simulink model "hcu_main_ADASwEPS"  (Simulink 8.2)
settings: Solver=FixedStepDiscrete  StartTime=0.0  StopTime=inf  FixedStep=0.001  RelTol=1e-3
PostLoadFcn:
  | , if any(exist('dsrtsu_mdlpostloadfcn', 'file') == [2, 3, 6]), try dsrtsu_mdlpostloadfcn('Execute', bdroot); catch fprintf('Error in PostLoadFcn (dsrtsu_mdlpostloadfcn) for model "%s":\n %s\n', bdroot, lasterr); end, end,
values from neighbouring files (symbols this model uses):
  C_TASK_1MS_S = (	C_TICK_TIME_S       )    [hcu_local_hdr.m]    (also in temp_ovrd_values.m = double(	0.001                  ))
  C_TICK_TIME_S = single(	0.005	    	)    [hcu_local_hdr.m]
  ENUM_EPSLFCSTATUS_ACTIVE = uint8(  2  )    [hcu_local_hdr.m]
  ENUM_EPSLFCSTATUS_TRANSITION = uint8(  3  )    [hcu_local_hdr.m]
  ENUM_EPSLKASTATUS_ACTIVE = uint8(  2  )    [hcu_local_hdr.m]
  ENUM_EPSMODEREQ_ANGLE = uint8(  1  )    [hcu_local_hdr.m]
  ENUM_EPSMODEREQ_INTERNAL = uint8(  0  )    [hcu_local_hdr.m]
  ENUM_EPSMODEREQ_TORQUE = uint8(  2  )    [hcu_local_hdr.m]
  ENUM_GEARPOSN_1ST = uint8(  1  )    [hcu_local_hdr.m]
  ENUM_GEARPOSN_2ND = uint8(  2  )    [hcu_local_hdr.m]
  ENUM_GEARPOSN_3RD = uint8(  3  )    [hcu_local_hdr.m]
  ENUM_GEARPOSN_4TH = uint8(  4  )    [hcu_local_hdr.m]
  ENUM_GEARPOSN_5TH = uint8(  5  )    [hcu_local_hdr.m]
  ENUM_GEARPOSN_6TH = uint8(  6  )    [hcu_local_hdr.m]
  ENUM_GEARPOSN_R = uint8(  7  )    [hcu_local_hdr.m]
  FALSE = boolean( 0 )    [hcu_local_hdr.m]
  TRUE = boolean( 1 )    [hcu_local_hdr.m]
undefined symbols (not defined in the file or in its folder): AISP_EPSCurrent_pct, AISP_TqASensorDelta_pct, AISP_TqBSensorDelta_pct, dHAL_IN, hal, INVALID_ABS1_TIMEOUT, INVALID_ABS2_TIMEOUT, INVALID_ABS3_TIMEOUT, INVALID_ABS4_TIMEOUT, INVALID_AC1_TIMEOUT, INVALID_ADASTORQ_REQ, INVALID_BCM1_TIMEOUT, INVALID_BCM2_TIMEOUT, INVALID_BOOSTER_VAC, INVALID_CSW1_TIMEOUT, INVALID_CUR_VEHDECE, INVALID_CURBRAKEDECE_REQ, INVALID_CURSTEERANG_REQ, INVALID_CURSTEERTQ_REQ, INVALID_ECM1_TIMEOUT, INVALID_ECM2_TIMEOUT, INVALID_ECM3_TIMEOUT, INVALID_ECM9_TIMEOUT, INVALID_ENG_TORQUE_FRICTIONAL, INVALID_ENG_TORQUE_INDICATED, INVALID_ENG_TORQUE_INDICATEDCOR, INVALID_ENG_TQ_MAX, INVALID_ENG_TQ_MIN, INVALID_EPAS2_TIMEOUT, INVALID_EPAS3_TIMEOUT, INVALID_EPB1_TIMEOUT, INVALID_EPS_BATTVOLT, INVALID_ESC_BATTVOLT, INVALID_GRADE, INVALID_HCU3_TIMEOUT, INVALID_HCU4_TIMEOUT, INVALID_HMI1_TIMEOUT, INVALID_HMI2_TIMEOUT, INVALID_LAT_ACC, INVALID_LONG_ACC, INVALID_MC_PRESSURE, INVALID_METER1_TIMEOUT, INVALID_METER3_TIMEOUT, INVALID_METER_VEHSPD, INVALID_ODO_METER, INVALID_OUTSIDE_TEMP, INVALID_PARKBRAKEBIND_STAT, INVALID_PEDALTQ_REQ, INVALID_SAS1_TIMEOUT, INVALID_SAS_ANGLE, INVALID_SHIFTER_POSN, INVALID_TCM1_TIMEOUT, INVALID_TCM2_TIMEOUT, INVALID_VCU1_TIMEOUT, INVALID_VCU2_TIMEOUT, INVALID_VEH_CRASH, INVALID_VEH_SPD, INVALID_WHEEL_SPD, INVALID_YAW_RATE, KHAL_MssgIdObj1_num ... (+8)
libraries: simulink x147, hcu_lib x38, rti1401lib_dio_type3 x4, rtimmsu_dsrtlib x3, app x1, rtiethernetudplib x1, rti1401lib_adc_type4 x1, rti1401lib_dac_type3 x1, inp x1, lidr x1, outp x1
(part 14 of 15)

== system hcu_main_ADASwEPS/dHAL_IN/HAL_IN_VCU/BO__1361_VCU2__8_VCU/ChecksumCalculation ==
  CAN1_Rx : Inport
  Add : Sum  Inputs=16
  Bitwise Operator : simulink/Logic and Bit Operations/Bitwise Operator  logicop=XOR  UseBitMask=off  NumInputPorts=2  BitMask=bin2dec('11011001')  BitMaskRealWorld=Stored Integer
  Bus Selector : BusSelector  OutputSignals=VCU2.RAW_Byte_1,VCU2.RAW_Byte_2,VCU2.RAW_Byte_3,VCU2.RAW_Byte_4,VCU2.RAW_Byte_5,VCU2.RAW_Byte_6,VCU2.RAW_Byte_7,VCU2.RAW_Byte_8,VCU2.VCU2_LifeCount
  Constant1 : Constant  Value=hex2dec('10')  OutDataTypeStr=uint8
  Constant2 : Constant  Value=hex2dec('ff')  OutDataTypeStr=uint8
  Data Type Conversion{,1..23} (24 alike) : DataTypeConversion  OutDataTypeStr=uint8
  Extract Bits{1,3,5,7,9,12,14} (7 alike) : simulink/Logic and Bit Operations/Extract Bits  bitsToExtract=Lower half  numBits=8  bitIdxRange=[0 7]  outScalingMode=Preserve fixed-point scaling
  Extract Bits{2,4,6,8,10..11,13,15} (8 alike) : simulink/Logic and Bit Operations/Extract Bits  bitsToExtract=Upper half  numBits=8  bitIdxRange=[0 7]  outScalingMode=Preserve fixed-point scaling
  Math Function : Math  Operator=mod  SaturateOnIntegerOverflow=on
  Shift Arithmetic{,1..7} (8 alike) : ArithShift  BitShiftNumber=4
  Message_Checksum : Outport
  wires:
  Bus Selector/1 -> Data Type Conversion/1  "<RAW_Byte_1>"
  Extract Bits2/1 -> Data Type Conversion1/1
  Extract Bits1/1 -> Data Type Conversion2/1
  Data Type Conversion1/1 -> Shift Arithmetic/1
  Data Type Conversion/1 -> Extract Bits2/1, Extract Bits1/1
  Extract Bits4/1 -> Data Type Conversion4/1
  Extract Bits3/1 -> Data Type Conversion5/1
  Data Type Conversion4/1 -> Shift Arithmetic1/1
  Data Type Conversion3/1 -> Extract Bits3/1, Extract Bits4/1
  Shift Arithmetic/1 -> Add/1
  Data Type Conversion2/1 -> Add/2
  Shift Arithmetic1/1 -> Add/3
  Data Type Conversion5/1 -> Add/4
  Bus Selector/2 -> Data Type Conversion3/1  "<RAW_Byte_2>"
  Extract Bits6/1 -> Data Type Conversion7/1
  Extract Bits5/1 -> Data Type Conversion8/1
  Data Type Conversion7/1 -> Shift Arithmetic2/1
  Data Type Conversion6/1 -> Extract Bits6/1, Extract Bits5/1
  Shift Arithmetic2/1 -> Add/5
  Data Type Conversion8/1 -> Add/6
  Bus Selector/3 -> Data Type Conversion6/1  "<RAW_Byte_3>"
  Extract Bits8/1 -> Data Type Conversion10/1
  Extract Bits7/1 -> Data Type Conversion11/1
  Data Type Conversion10/1 -> Shift Arithmetic3/1
  Data Type Conversion9/1 -> Extract Bits7/1, Extract Bits8/1
  Shift Arithmetic3/1 -> Add/7
  Data Type Conversion11/1 -> Add/8
  Bus Selector/4 -> Data Type Conversion9/1  "<RAW_Byte_4>"
  Extract Bits10/1 -> Data Type Conversion12/1
  Extract Bits9/1 -> Data Type Conversion13/1
  Data Type Conversion12/1 -> Shift Arithmetic4/1
  Data Type Conversion14/1 -> Extract Bits10/1, Extract Bits9/1
  Shift Arithmetic4/1 -> Add/9
  Data Type Conversion13/1 -> Add/10
  Bus Selector/5 -> Data Type Conversion14/1  "<RAW_Byte_5>"
  Extract Bits11/1 -> Data Type Conversion15/1
  Extract Bits12/1 -> Data Type Conversion16/1
  Data Type Conversion15/1 -> Shift Arithmetic5/1
  Data Type Conversion17/1 -> Extract Bits12/1, Extract Bits11/1
  Shift Arithmetic5/1 -> Add/11
  Data Type Conversion16/1 -> Add/12
  Bus Selector/6 -> Data Type Conversion17/1  "<RAW_Byte_6>"
  Extract Bits13/1 -> Data Type Conversion18/1
  Extract Bits14/1 -> Data Type Conversion19/1
  Data Type Conversion18/1 -> Shift Arithmetic6/1
  Data Type Conversion20/1 -> Extract Bits13/1, Extract Bits14/1
  Shift Arithmetic6/1 -> Add/13
  Data Type Conversion19/1 -> Add/14
  Bus Selector/7 -> Data Type Conversion20/1  "<RAW_Byte_7>"
  Extract Bits15/1 -> Data Type Conversion21/1
  Data Type Conversion21/1 -> Shift Arithmetic7/1
  Data Type Conversion23/1 -> Extract Bits15/1
  Shift Arithmetic7/1 -> Add/15
  Bus Selector/8 -> Data Type Conversion23/1  "<RAW_Byte_8>"
  Data Type Conversion22/1 -> Add/16
  Add/1 -> Bitwise Operator/1
  Constant2/1 -> Bitwise Operator/2
  Bitwise Operator/1 -> Math Function/1
  Constant1/1 -> Math Function/2
  Math Function/1 -> Message_Checksum/1
  CAN1_Rx/1 -> Bus Selector/1
  Bus Selector/9 -> Data Type Conversion22/1  "<VCU2_LifeCount>"

== system hcu_main_ADASwEPS/dHAL_IN/dHAL_IN_ABS/BO_864_ABS2_8_ABS/ChecksumCalculation ==
  CAN1_Rx : Inport
  Add : Sum  Inputs=16
  Bitwise Operator : simulink/Logic and Bit Operations/Bitwise Operator  logicop=XOR  UseBitMask=off  NumInputPorts=2  BitMask=bin2dec('11011001')  BitMaskRealWorld=Stored Integer
  Bus Selector : BusSelector  OutputSignals=ABS2.RAW_Byte_1,ABS2.RAW_Byte_2,ABS2.RAW_Byte_3,ABS2.RAW_Byte_4,ABS2.RAW_Byte_5,ABS2.RAW_Byte_6,ABS2.RAW_Byte_7,ABS2.RAW_Byte_8
  Constant : Constant  Value=uint8(2)
  Constant1 : Constant  Value=hex2dec('10')  OutDataTypeStr=uint8
  Constant2 : Constant  Value=hex2dec('ff')  OutDataTypeStr=uint8
  Data Type Conversion{,1..21,23} (23 alike) : DataTypeConversion  OutDataTypeStr=uint8
  Extract Bits{1,3,5,7,9,12,14} (7 alike) : simulink/Logic and Bit Operations/Extract Bits  bitsToExtract=Lower half  numBits=8  bitIdxRange=[0 7]  outScalingMode=Preserve fixed-point scaling
  Extract Bits{2,4,6,8,10..11,13,15} (8 alike) : simulink/Logic and Bit Operations/Extract Bits  bitsToExtract=Upper half  numBits=8  bitIdxRange=[0 7]  outScalingMode=Preserve fixed-point scaling
  Math Function : Math  Operator=mod  SaturateOnIntegerOverflow=on
  Shift Arithmetic{,1..7} (8 alike) : ArithShift  BitShiftNumber=4
  Message_Checksum : Outport
  wires:
  Bus Selector/1 -> Data Type Conversion/1  "<RAW_Byte_1>"
  Extract Bits2/1 -> Data Type Conversion1/1
  Extract Bits1/1 -> Data Type Conversion2/1
  Data Type Conversion1/1 -> Shift Arithmetic/1
  Data Type Conversion/1 -> Extract Bits2/1, Extract Bits1/1
  Extract Bits4/1 -> Data Type Conversion4/1
  Extract Bits3/1 -> Data Type Conversion5/1
  Data Type Conversion4/1 -> Shift Arithmetic1/1
  Data Type Conversion3/1 -> Extract Bits3/1, Extract Bits4/1
  Shift Arithmetic/1 -> Add/1
  Data Type Conversion2/1 -> Add/2
  Shift Arithmetic1/1 -> Add/3
  Data Type Conversion5/1 -> Add/4
  Bus Selector/2 -> Data Type Conversion3/1  "<RAW_Byte_2>"
  Extract Bits6/1 -> Data Type Conversion7/1
  Extract Bits5/1 -> Data Type Conversion8/1
  Data Type Conversion7/1 -> Shift Arithmetic2/1
  Data Type Conversion6/1 -> Extract Bits6/1, Extract Bits5/1
  Shift Arithmetic2/1 -> Add/5
  Data Type Conversion8/1 -> Add/6
  Bus Selector/3 -> Data Type Conversion6/1  "<RAW_Byte_3>"
  Extract Bits8/1 -> Data Type Conversion10/1
  Extract Bits7/1 -> Data Type Conversion11/1
  Data Type Conversion10/1 -> Shift Arithmetic3/1
  Data Type Conversion9/1 -> Extract Bits7/1, Extract Bits8/1
  Shift Arithmetic3/1 -> Add/7
  Data Type Conversion11/1 -> Add/8
  Bus Selector/4 -> Data Type Conversion9/1  "<RAW_Byte_4>"
  Extract Bits10/1 -> Data Type Conversion12/1
  Extract Bits9/1 -> Data Type Conversion13/1
  Data Type Conversion12/1 -> Shift Arithmetic4/1
  Data Type Conversion14/1 -> Extract Bits10/1, Extract Bits9/1
  Shift Arithmetic4/1 -> Add/9
  Data Type Conversion13/1 -> Add/10
  Bus Selector/5 -> Data Type Conversion14/1  "<RAW_Byte_5>"
  Extract Bits11/1 -> Data Type Conversion15/1
  Extract Bits12/1 -> Data Type Conversion16/1
  Data Type Conversion15/1 -> Shift Arithmetic5/1
  Data Type Conversion17/1 -> Extract Bits12/1, Extract Bits11/1
  Shift Arithmetic5/1 -> Add/11
  Data Type Conversion16/1 -> Add/12
  Bus Selector/6 -> Data Type Conversion17/1  "<RAW_Byte_6>"
  Extract Bits13/1 -> Data Type Conversion18/1
  Extract Bits14/1 -> Data Type Conversion19/1
  Data Type Conversion18/1 -> Shift Arithmetic6/1
  Data Type Conversion20/1 -> Extract Bits13/1, Extract Bits14/1
  Shift Arithmetic6/1 -> Add/13
  Data Type Conversion19/1 -> Add/14
  Bus Selector/7 -> Data Type Conversion20/1  "<RAW_Byte_7>"
  Extract Bits15/1 -> Data Type Conversion21/1
  Data Type Conversion21/1 -> Shift Arithmetic7/1
  Data Type Conversion23/1 -> Extract Bits15/1
  Shift Arithmetic7/1 -> Add/15
  Bus Selector/8 -> Data Type Conversion23/1  "<RAW_Byte_8>"
  Constant/1 -> Add/16
  Add/1 -> Bitwise Operator/1
  Constant2/1 -> Bitwise Operator/2
  Bitwise Operator/1 -> Math Function/1
  Constant1/1 -> Math Function/2
  Math Function/1 -> Message_Checksum/1
  CAN1_Rx/1 -> Bus Selector/1

== system hcu_main_ADASwEPS/dHAL_IN/dHAL_IN_EPAS/BO__1365_EPAS3__8_EPAS/ChecksumCalculation ==
  EPAS3_LifeCount : Inport
  CAN1_Rx : Inport  Port=2
  Bitwise Operator1 : simulink/Logic and Bit Operations/Bitwise Operator  logicop=XOR  UseBitMask=off  NumInputPorts=7  BitMask=bin2dec('11011001')  BitMaskRealWorld=Stored Integer
  Bitwise Operator2 : simulink/Logic and Bit Operations/Bitwise Operator  logicop=XOR  UseBitMask=off  NumInputPorts=3  BitMask=bin2dec('11011001')  BitMaskRealWorld=Stored Integer
  Bus Selector : BusSelector  OutputSignals=EPAS3.RAW_Byte_1,EPAS3.RAW_Byte_2,EPAS3.RAW_Byte_3,EPAS3.RAW_Byte_4,EPAS3.RAW_Byte_5,EPAS3.RAW_Byte_6,EPAS3.RAW_Byte_7
  Data Type Conversion{1..10} (10 alike) : DataTypeConversion  OutDataTypeStr=uint8
  Extract Bits5 : simulink/Logic and Bit Operations/Extract Bits  bitsToExtract=Lower half  numBits=8  bitIdxRange=[0 7]  outScalingMode=Preserve fixed-point scaling
  Extract Bits6 : simulink/Logic and Bit Operations/Extract Bits  bitsToExtract=Upper half  numBits=8  bitIdxRange=[0 7]  outScalingMode=Preserve fixed-point scaling
  Shift Arithmetic2 : ArithShift  BitShiftNumber=4
  Message_Checksum : Outport
  wires:
  [CAN1_Rx] -> Bus Selector/1
  CAN1_Rx/1 -> [CAN1_Rx]
  Bitwise Operator2/1 -> Message_Checksum/1
  EPAS3_LifeCount/1 -> Data Type Conversion10/1
  Data Type Conversion8/1 -> Bitwise Operator2/2
  Shift Arithmetic2/1 -> Bitwise Operator2/1
  Bitwise Operator1/1 -> Extract Bits5/1, Extract Bits6/1
  Data Type Conversion9/1 -> Bitwise Operator1/4
  Data Type Conversion6/1 -> Bitwise Operator1/3
  Data Type Conversion3/1 -> Bitwise Operator1/2
  Data Type Conversion1/1 -> Bitwise Operator1/1
  Bus Selector/1 -> Data Type Conversion1/1  "<RAW_Byte_1>"
  Bus Selector/4 -> Data Type Conversion9/1  "<RAW_Byte_4>"
  Bus Selector/3 -> Data Type Conversion6/1  "<RAW_Byte_3>"
  Data Type Conversion7/1 -> Shift Arithmetic2/1
  Extract Bits5/1 -> Data Type Conversion8/1
  Extract Bits6/1 -> Data Type Conversion7/1
  Bus Selector/2 -> Data Type Conversion3/1  "<RAW_Byte_2>"
  Data Type Conversion2/1 -> Bitwise Operator1/5
  Data Type Conversion4/1 -> Bitwise Operator1/6
  Data Type Conversion5/1 -> Bitwise Operator1/7
  Bus Selector/5 -> Data Type Conversion2/1  "<RAW_Byte_5>"
  Bus Selector/6 -> Data Type Conversion4/1  "<RAW_Byte_6>"
  Bus Selector/7 -> Data Type Conversion5/1  "<RAW_Byte_7>"
  Data Type Conversion10/1 -> Bitwise Operator2/3

== system hcu_main_ADASwEPS/dHAL_IN/dHAL_IN_EPAS/BO__922_SAS1__8_EPAS/ChecksumCalculation ==
  SAS_MsgCount : Inport
  CAN1_Rx : Inport  Port=2
  Bitwise Operator1 : simulink/Logic and Bit Operations/Bitwise Operator  logicop=XOR  UseBitMask=off  NumInputPorts=4  BitMask=bin2dec('11011001')  BitMaskRealWorld=Stored Integer
  Bitwise Operator2 : simulink/Logic and Bit Operations/Bitwise Operator  logicop=XOR  UseBitMask=off  NumInputPorts=3  BitMask=bin2dec('11011001')  BitMaskRealWorld=Stored Integer
  Bus Selector : BusSelector  OutputSignals=SAS1.RAW_Byte_1,SAS1.RAW_Byte_2,SAS1.RAW_Byte_3,SAS1.RAW_Byte_4
  Data Type Conversion{1..3,6..9} (7 alike) : DataTypeConversion  OutDataTypeStr=uint8
  Extract Bits5 : simulink/Logic and Bit Operations/Extract Bits  bitsToExtract=Lower half  numBits=8  bitIdxRange=[0 7]  outScalingMode=Preserve fixed-point scaling
  Extract Bits6 : simulink/Logic and Bit Operations/Extract Bits  bitsToExtract=Upper half  numBits=8  bitIdxRange=[0 7]  outScalingMode=Preserve fixed-point scaling
  Shift Arithmetic2 : ArithShift  BitShiftNumber=4
  Message_Checksum : Outport
  wires:
  Bus Selector/2 -> Data Type Conversion3/1  "<RAW_Byte_2>"
  Extract Bits6/1 -> Data Type Conversion7/1
  Extract Bits5/1 -> Data Type Conversion8/1
  Data Type Conversion7/1 -> Shift Arithmetic2/1
  Bus Selector/3 -> Data Type Conversion6/1  "<RAW_Byte_3>"
  Bus Selector/4 -> Data Type Conversion9/1  "<RAW_Byte_4>"
  Bus Selector/1 -> Data Type Conversion1/1  "<RAW_Byte_1>"
  Data Type Conversion1/1 -> Bitwise Operator1/1
  Data Type Conversion3/1 -> Bitwise Operator1/2
  Data Type Conversion6/1 -> Bitwise Operator1/3
  Data Type Conversion9/1 -> Bitwise Operator1/4
  Bitwise Operator1/1 -> Extract Bits6/1, Extract Bits5/1
  Shift Arithmetic2/1 -> Bitwise Operator2/1
  Data Type Conversion8/1 -> Bitwise Operator2/2
  SAS_MsgCount/1 -> Data Type Conversion2/1
  Bitwise Operator2/1 -> Message_Checksum/1
  CAN1_Rx/1 -> Bus Selector/1
  Data Type Conversion2/1 -> Bitwise Operator2/3

== system hcu_main_ADASwEPS/dHAL_IN/dHAL_IN_EPAS/BO__926_EPAS2__8_EPAS/ChecksumCalculation ==
  SAS_MsgCount : Inport
  CAN1_Rx : Inport  Port=2
  Bitwise Operator1 : simulink/Logic and Bit Operations/Bitwise Operator  logicop=XOR  UseBitMask=off  NumInputPorts=5  BitMask=bin2dec('11011001')  BitMaskRealWorld=Stored Integer
  Bitwise Operator2 : simulink/Logic and Bit Operations/Bitwise Operator  logicop=XOR  UseBitMask=off  NumInputPorts=3  BitMask=bin2dec('11011001')  BitMaskRealWorld=Stored Integer
  Bus Selector : BusSelector  OutputSignals=EPAS2.RAW_Byte_1,EPAS2.RAW_Byte_2,EPAS2.RAW_Byte_3,EPAS2.RAW_Byte_4,EPAS2.RAW_Byte_5
  Data Type Conversion{1..4,6..9} (8 alike) : DataTypeConversion  OutDataTypeStr=uint8
  Extract Bits5 : simulink/Logic and Bit Operations/Extract Bits  bitsToExtract=Lower half  numBits=8  bitIdxRange=[0 7]  outScalingMode=Preserve fixed-point scaling
  Extract Bits6 : simulink/Logic and Bit Operations/Extract Bits  bitsToExtract=Upper half  numBits=8  bitIdxRange=[0 7]  outScalingMode=Preserve fixed-point scaling
  Shift Arithmetic2 : ArithShift  BitShiftNumber=4
  Message_Checksum : Outport
  wires:
  Bus Selector/2 -> Data Type Conversion3/1  "<RAW_Byte_2>"
  Extract Bits6/1 -> Data Type Conversion7/1
  Extract Bits5/1 -> Data Type Conversion8/1
  Data Type Conversion7/1 -> Shift Arithmetic2/1
  Bus Selector/3 -> Data Type Conversion6/1  "<RAW_Byte_3>"
  Bus Selector/4 -> Data Type Conversion9/1  "<RAW_Byte_4>"
  Bus Selector/1 -> Data Type Conversion1/1  "<RAW_Byte_1>"
  Data Type Conversion1/1 -> Bitwise Operator1/1
  Data Type Conversion3/1 -> Bitwise Operator1/2
  Data Type Conversion6/1 -> Bitwise Operator1/3
  Data Type Conversion9/1 -> Bitwise Operator1/4
  Bitwise Operator1/1 -> Extract Bits5/1, Extract Bits6/1
  Shift Arithmetic2/1 -> Bitwise Operator2/1
  Data Type Conversion8/1 -> Bitwise Operator2/2
  SAS_MsgCount/1 -> Data Type Conversion4/1
  Bitwise Operator2/1 -> Message_Checksum/1
  CAN1_Rx/1 -> [CAN1_Rx]
  [CAN1_Rx] -> Bus Selector/1
  Bus Selector/5 -> Data Type Conversion2/1  "<RAW_Byte_5>"
  Data Type Conversion2/1 -> Bitwise Operator1/5
  Data Type Conversion4/1 -> Bitwise Operator2/3

== system hcu_main_ADASwEPS/EPSS/EPSS/AngleMode/Angle2Torque/Hysteresis (higher limit) ==
  Input : Inport
  Switch_on_point : Inport  Port=2
  Switch_off_point : Inport  Port=3
  Data Type Conversion : DataTypeConversion
  Logical Operator1 : Logic  AllPortsSameDT=off  OutDataTypeStr=boolean
  Logical Operator2 : Logic  Operator=NOT  AllPortsSameDT=off  OutDataTypeStr=boolean
  Logical Operator3 : Logic  Operator=OR  AllPortsSameDT=off  OutDataTypeStr=boolean
  Relational Operator : RelationalOperator  OutDataTypeStr=boolean
  Relational Operator1 : RelationalOperator  Operator=<=  OutDataTypeStr=boolean
  Unit Delay : UnitDelay  SampleTime=-1
  Output : Outport
  wires:
  Switch_on_point/1 -> Relational Operator/2
  Switch_off_point/1 -> Relational Operator1/2
  Logical Operator2/1 -> Logical Operator1/2
  Logical Operator1/1 -> Unit Delay/1, Data Type Conversion/1
  Unit Delay/1 -> Logical Operator3/1
  Input/1 -> Relational Operator/1, Relational Operator1/1
  Relational Operator/1 -> Logical Operator3/2
  Logical Operator3/1 -> Logical Operator1/1
  Relational Operator1/1 -> Logical Operator2/1
  Data Type Conversion/1 -> Output/1

== system hcu_main_ADASwEPS/EPSS/EPSS/AngleMode/Angle2Torque/InverseAssistTable ==
  VEPSS_MotPWMReqAngle_pct : Inport
  VDINR_VehSpd_kph : Inport  Port=2
  MEPSS_EPSMotPWMRescalingInv_pct : Lookup  InputValues=[-250 -3 0 3 250]  Table=[-100 -3 0 3 100]  LookUpMeth=Interpolation-Use End Values
      settings: AttributesFormatString="Input=\"%<InputValues>\"\\nOutput=\"%<Table>\""
  MEPSS_TqAssistPWM_pct : Lookup  InputValues="[-100\t-95\t-90\t-85\t-80\t-75\t-70\t-65\t-60\t-55\t-50\t-45\t-40\t-35\t-30\t-25\t-20\t-15\t-10\t-5\t0\t5\t10\t15\t20\t25\t30\t35\t40\t45\t50\t55\t60\t65\t70\t75\t80\t85\t90\t95\t100]"  Table=[-10:0.5:10]  LookUpMeth=Interpolation-Use End Values
      settings: AttributesFormatString="Input=\"%<InputValues>\"\\nOutput=\"%<Table>\""
  MEPSS_VehSpdPWMMult_rat : Lookup  InputValues=[-100 -80 -60 -40 -20 -10 0 10 20 40 60 80 100]  Table=[1 1 1 1 1 1 1 1 1 1 1 1 1]  LookUpMeth=Interpolation-Use End Values
      settings: AttributesFormatString="Input=\"%<InputValues>\"\\nOutput=\"%<Table>\""
  Product : Product  Inputs=*/
  VEPSS_StrWhlTqReqAngRaw_Nm : Outport
  wires:
  MEPSS_EPSMotPWMRescalingInv_pct/1 -> Product/1
  VEPSS_MotPWMReqAngle_pct/1 -> MEPSS_EPSMotPWMRescalingInv_pct/1
  VDINR_VehSpd_kph/1 -> MEPSS_VehSpdPWMMult_rat/1
  MEPSS_VehSpdPWMMult_rat/1 -> Product/2
  Product/1 -> MEPSS_TqAssistPWM_pct/1
  MEPSS_TqAssistPWM_pct/1 -> VEPSS_StrWhlTqReqAngRaw_Nm/1  "VEPSS_StrWhlTqReqAngRaw_Nm"

== system hcu_main_ADASwEPS/EPSS/EPSS/AngleMode/Angle2Torque/Rate_Limit ==
  Data_Input : Inport
  Rising_Rate : Inport  Port=2
  Falling_Rate : Inport  Port=3
  Initial_condition : Inport  Port=4
  Enable : EnablePort  StatesWhenEnabling=reset
  RateLimiter : Subsystem
  Data_Output : Outport  OutputWhenDisabled=reset  InitialOutput=[0]
  wires:
  RateLimiter/1(Data_Output) -> Data_Output/1
  Data_Input/1 -> RateLimiter/1(Data_Input)
  Initial_condition/1 -> RateLimiter/4(Initial_Condition)
  Falling_Rate/1 -> RateLimiter/3(Falling Rate)
  Rising_Rate/1 -> RateLimiter/2(Rising Rate)

== system hcu_main_ADASwEPS/EPSS/EPSS/EPSTest/SignalPlayer/Timer ==
  Enable : EnablePort  StatesWhenEnabling=reset
  C_TASK_1MS_S : Constant  Value=C_TASK_1MS_S
  Sum : Sum  Inputs=|++
  Unit Delay : UnitDelay  SampleTime=-1
  Unit Delay1 : UnitDelay  SampleTime=-1
  SineTime_s : Outport  OutputWhenDisabled=reset  InitialOutput=[0]
  wires:
  Unit Delay1/1 -> Sum/1
  Unit Delay/1 -> Sum/2
  Sum/1 -> SineTime_s/1, Unit Delay/1  "SineTime_s"
  C_TASK_1MS_S/1 -> Unit Delay1/1

== system hcu_main_ADASwEPS/EPSS/EPSS/EPSTest/SignalPlayer/Timer1 ==
  Enable : EnablePort  StatesWhenEnabling=reset
  C_TASK_1MS_S : Constant  Value=C_TASK_1MS_S
  Sum : Sum  Inputs=|++
  Unit Delay : UnitDelay  SampleTime=-1
  Unit Delay1 : UnitDelay  SampleTime=-1
  SineTime_s : Outport  OutputWhenDisabled=reset  InitialOutput=[0]
  wires:
  C_TASK_1MS_S/1 -> Unit Delay1/1
  Sum/1 -> Unit Delay/1, SineTime_s/1  "SineTime_s"
  Unit Delay/1 -> Sum/2
  Unit Delay1/1 -> Sum/1

== system hcu_main_ADASwEPS/OSP/OSP/CheckSum Calculation/Byte0/SAS_Angle_cvt ==
  value : Inport
  Add : Sum  Inputs=+-
  Data Type Conversion : DataTypeConversion  OutDataTypeStr=uint32  RndMeth=Nearest
  Divide : Product  Inputs=*/
  gain : Constant  Value=single(gain)  OutDataTypeStr=single
  offset : Constant  Value=single(offset)  OutDataTypeStr=single
  raw32 : Outport
  wires:
  Data Type Conversion/1 -> raw32/1
  gain/1 -> Divide/2
  Add/1 -> Divide/1
  Divide/1 -> Data Type Conversion/1
  offset/1 -> Add/2
  value/1 -> Add/1

== system hcu_main_ADASwEPS/OSP/OSP/CheckSum Calculation1/Byte0/Elect_PWR_Consumpt_cvt ==
  value : Inport
  Add : Sum  Inputs=+-
  Data Type Conversion : DataTypeConversion  OutDataTypeStr=uint32  RndMeth=Nearest
  Divide : Product  Inputs=*/
  gain : Constant  Value=single(gain)  OutDataTypeStr=single
  offset : Constant  Value=single(offset)  OutDataTypeStr=single
  raw32 : Outport
  wires:
  value/1 -> Add/1
  offset/1 -> Add/2
  Divide/1 -> Data Type Conversion/1
  Add/1 -> Divide/1
  gain/1 -> Divide/2
  Data Type Conversion/1 -> raw32/1

== system hcu_main_ADASwEPS/OSP/OSP/CheckSum Calculation1/Byte2/Steering_Torque_cvt ==
  value : Inport
  Add : Sum  Inputs=+-
  Data Type Conversion : DataTypeConversion  OutDataTypeStr=uint32  RndMeth=Nearest
  Divide : Product  Inputs=*/
  gain : Constant  Value=single(gain)  OutDataTypeStr=single
  offset : Constant  Value=single(offset)  OutDataTypeStr=single
  raw32 : Outport
  wires:
  Data Type Conversion/1 -> raw32/1
  gain/1 -> Divide/2
  Add/1 -> Divide/1
  Divide/1 -> Data Type Conversion/1
  offset/1 -> Add/2
  value/1 -> Add/1

== system hcu_main_ADASwEPS/OSP/OSP/CheckSum Calculation1/Byte3/R_SAS_Angle_cvt ==
  value : Inport
  Add : Sum  Inputs=+-
  Data Type Conversion : DataTypeConversion  OutDataTypeStr=uint32  RndMeth=Nearest
  Divide : Product  Inputs=*/
  gain : Constant  Value=single(gain)  OutDataTypeStr=single
  offset : Constant  Value=single(offset)  OutDataTypeStr=single
  raw32 : Outport
  wires:
  Data Type Conversion/1 -> raw32/1
  gain/1 -> Divide/2
  Add/1 -> Divide/1
  Divide/1 -> Data Type Conversion/1
  offset/1 -> Add/2
  value/1 -> Add/1

== system hcu_main_ADASwEPS/OSP/OSP/CheckSum Calculation2/Byte0/CurStrAngReq_cvt ==
  value : Inport
  Add : Sum  Inputs=+-
  Data Type Conversion : DataTypeConversion  OutDataTypeStr=uint32  RndMeth=Nearest
  Divide : Product  Inputs=*/
  gain : Constant  Value=single(gain)  OutDataTypeStr=single
  offset : Constant  Value=single(offset)  OutDataTypeStr=single
  raw32 : Outport
  wires:
  value/1 -> Add/1
  offset/1 -> Add/2
  Divide/1 -> Data Type Conversion/1
  Add/1 -> Divide/1
  gain/1 -> Divide/2
  Data Type Conversion/1 -> raw32/1

== system hcu_main_ADASwEPS/OSP/OSP/CheckSum Calculation2/Byte4/CurStrTqReq_cvt ==
  value : Inport
  Add : Sum  Inputs=+-
  Data Type Conversion : DataTypeConversion  OutDataTypeStr=uint32  RndMeth=Nearest
  Divide : Product  Inputs=*/
  gain : Constant  Value=single(gain)  OutDataTypeStr=single
  offset : Constant  Value=single(offset)  OutDataTypeStr=single
  raw32 : Outport
  wires:
  Data Type Conversion/1 -> raw32/1
  gain/1 -> Divide/2
  Add/1 -> Divide/1
  Divide/1 -> Data Type Conversion/1
  offset/1 -> Add/2
  value/1 -> Add/1

== system hcu_main_ADASwEPS/OSP/OSP/CheckSum Calculation2/Byte5/EPSBattVolt_cvt ==
  value : Inport
  Add : Sum  Inputs=+-
  Data Type Conversion : DataTypeConversion  OutDataTypeStr=uint32  RndMeth=Nearest
  Divide : Product  Inputs=*/
  gain : Constant  Value=single(gain)  OutDataTypeStr=single
  offset : Constant  Value=single(offset)  OutDataTypeStr=single
  raw32 : Outport
  wires:
  value/1 -> Add/1
  offset/1 -> Add/2
  Divide/1 -> Data Type Conversion/1
  Add/1 -> Divide/1
  gain/1 -> Divide/2
  Data Type Conversion/1 -> raw32/1

== system hcu_main_ADASwEPS/RTI Data/RTI Data Store/RTI Data Store/RTI Data Store/RTI Data Store ==

== system hcu_main_ADASwEPS/dHAL_IN/HAL_IN_RadObjDecoder/RObjectPackFrame/RObjects_Decoder_v2/CheckIDs ==
  Status : Inport
  ID : Inport  Port=2
  R_Objects_in : Inport  Port=3  OutDataTypeStr=Bus: R_Objects
  CAN_RAW_Deco : Stateflow chart  TreatAsAtomicUnit=on
  R_Objects_out : Outport  OutDataTypeStr=Bus: R_Objects
  ParseFrame : Outport  Port=2
  wires:
  CAN_RAW_Deco/1(R_Objects_out) -> R_Objects_out/1
  R_Objects_in/1 -> CAN_RAW_Deco/3(R_Objects_in)
  CAN_RAW_Deco/2(ParseFrames()) -> ParseFrame/1
  ID/1 -> CAN_RAW_Deco/2(ID)
  Status/1 -> CAN_RAW_Deco/1(Status)

== system hcu_main_ADASwEPS/dHAL_IN/HAL_IN_RadObjDecoder/RObjectPackFrame/RObjects_Decoder_v2/ParseFrames ==
  R_Objects_in : Inport  OutDataTypeStr=Bus: R_Objects
  Byte1 : Inport  Port=2
  Byte2 : Inport  Port=3
  Byte3 : Inport  Port=4
  Byte4 : Inport  Port=5
  Byte5 : Inport  Port=6
  Byte6 : Inport  Port=7
  Byte7 : Inport  Port=8
  Byte8 : Inport  Port=9
  Trigger : TriggerPort  TriggerType=function-call  PortDimensions=1
  MATLAB Function : MATLAB Function  TreatAsAtomicUnit=on
  R_Objects_out : Outport  OutDataTypeStr=Bus: R_Objects
  wires:
  MATLAB Function/1(R_Objects_out) -> R_Objects_out/1
  R_Objects_in/1 -> MATLAB Function/1(R_Objects_in)
  Byte2/1 -> MATLAB Function/3(Byte2)
  Byte3/1 -> MATLAB Function/4(Byte3)
  Byte4/1 -> MATLAB Function/5(Byte4)
  Byte8/1 -> MATLAB Function/9(Byte8)
  Byte6/1 -> MATLAB Function/7(Byte6)
  Byte5/1 -> MATLAB Function/6(Byte5)
  Byte1/1 -> MATLAB Function/2(Byte1)
  Byte7/1 -> MATLAB Function/8(Byte7)

== system hcu_main_ADASwEPS/EPSS/EPSS/AngleMode/Angle2Torque/Rate_Limit/RateLimiter ==
  Data_Input : Inport
  Rising Rate : Inport  Port=2
  Falling Rate : Inport  Port=3
  Initial_Condition : Inport  Port=4
  Chart : Stateflow chart  TreatAsAtomicUnit=on
  Constant : Constant  Value=C_TASK_1MS_S
  Constant1 : Constant  Value=C_TASK_1MS_S
  Constant4 : Constant
  Constant5 : Constant
  Data Type Conversion : DataTypeConversion  OutDataTypeStr=boolean
  Data Type Conversion1 : DataTypeConversion  OutDataTypeStr=boolean
  Product{1..4} (4 alike) : Product  Inputs=*/  RndMeth=Zero
  Relational Operator : RelationalOperator  Operator=>  OutDataTypeStr=boolean
  Relational Operator1 : RelationalOperator  Operator=<  OutDataTypeStr=boolean
  Saturation : Subsystem
  Sum1 : Sum  Inputs=|++
  Switch1 : Switch  Threshold=0.5
  Unit Delay1 : UnitDelay  SampleTime=-1
  Data_Output : Outport
  wires:
  Relational Operator1/1 -> Data Type Conversion/1
  Relational Operator/1 -> Data Type Conversion1/1
  Data_Input/1 -> Relational Operator/1, Relational Operator1/1, Chart/3(Data_in)
  Product3/1 -> Product1/2
  Product4/1 -> Product2/2
  Product1/1 -> Chart/4(increase_tou)
  Product2/1 -> Chart/5(decrease_tou)
  Data Type Conversion/1 -> Chart/2(decrease)
  Data Type Conversion1/1 -> Chart/1(increase)
  Chart/2(tou) -> Sum1/1
  Saturation/1(out) -> Switch1/3
  Chart/3(Min) -> Saturation/2(min)
  Chart/4(Max) -> Saturation/3(max)
  Chart/1(Initial) -> Switch1/2
  Initial_Condition/1 -> Switch1/1
  Constant/1 -> Product3/2
  Constant4/1 -> Product3/1
  Constant1/1 -> Product4/2
  Constant5/1 -> Product4/1
  Switch1/1 -> Data_Output/1, Unit Delay1/1
  Rising Rate/1 -> Product1/1
  Falling Rate/1 -> Product2/1
  Sum1/1 -> Saturation/1(in)
  Unit Delay1/1 -> Sum1/2, Relational Operator/2, Relational Operator1/2

== system hcu_main_ADASwEPS/EPSS/EPSS/AngleMode/Angle2Torque/Rate_Limit/RateLimiter/Saturation ==
  in : Inport
  min : Inport  Port=2
  max : Inport  Port=3
  MinMax : MinMax  Function=max  Inputs=2  ZeroCross=off  SaturateOnIntegerOverflow=on  InputSameDT=on
  MinMax1 : MinMax  Inputs=2  ZeroCross=off  SaturateOnIntegerOverflow=on  InputSameDT=on
  out : Outport
  wires:
  MinMax1/1 -> out/1
  max/1 -> MinMax1/2
  min/1 -> MinMax/2
  in/1 -> MinMax/1
  MinMax/1 -> MinMax1/1

== stateflow chart Scheduler ==
  settings: sampleTime=0.003125
  (default) -> (junction 19)
  (junction 19) -> (junction 20) : {
      | b1ms_count = b1ms_count +1; ...
      | b5ms_count = b5ms_count +1; ...
      | b10ms_count=b10ms_count+1; ...
      | b50ms_count=b50ms_count+1; ...
      | b100ms_count=b100ms_count+1; ...
      | b200ms_count=b200ms_count+1; ...
      | //trig_LIDR; ...
      | trig_Hw_In; ...
      | trig_ISP; ...
      | trig_EPSS; ...
      | trig_OSP; ...
      | trig_Hw_Out; ...
      | }
  (junction 20) -> (junction 21) [order 1] : [b1ms_count == 1]
  (junction 20) -> (junction 22) [order 2]
  (junction 21) -> (junction 23) : /*1ms*/
      | {
      | b1ms_count = 0; ...
      | }
  (junction 23) -> (junction 22)
  (junction 22) -> (junction 24)
  (junction 24) -> (junction 25) [order 1] : [b5ms_count == 5]
  (junction 24) -> (junction 26) [order 2]
  (junction 25) -> (junction 27) : /*5ms*/
      | {
      | b5ms_count = 0; ...
      | trig_HAL_In; ...
      | trig_INP; ...
      | trig_APP; ...
      | trig_OUTP; ...
      | }
  (junction 27) -> (junction 26)
  (junction 26) -> (junction 28)
  (junction 28) -> (junction 29) [order 1] : [b10ms_count == 10]
  (junction 28) -> (junction 30) [order 2]
  (junction 29) -> (junction 31) : /*10ms*/
      | {
      | b10ms_count = 0;
      | }
  (junction 31) -> (junction 30)
  (junction 30) -> (junction 32)
  (junction 32) -> (junction 33) [order 1] : [b50ms_count == 50]
  (junction 32) -> (junction 34) [order 2]
  (junction 33) -> (junction 35) : /*50ms*/
      | {
      | b50ms_count = 0;
      | }
  (junction 35) -> (junction 34)
  (junction 34) -> (junction 36)
  (junction 36) -> (junction 37) [order 1] : [b100ms_count == 100]
  (junction 36) -> (junction 38) [order 2]
  (junction 37) -> (junction 39) : /*100ms*/
      | {
      | b100ms_count = 0;
      | }
  (junction 39) -> (junction 38)
  (junction 38) -> (junction 40)
  (junction 40) -> (junction 41) [order 1] : [b200ms_count == 200]
  (junction 40) -> (junction 42) [order 2]
  (junction 41) -> (junction 43) : /*200ms*/
      | {
      | b200ms_count = 0;
      | }
  (junction 43) -> (junction 42)
  data: b10ms_count local uint8; b5ms_count local uint8; b50ms_count local uint8; b100ms_count local uint8; b200ms_count local uint8; b1ms_count local uint8
  events: trig_Hw_In output FUNCTION_CALL_EVENT; trig_ISP output FUNCTION_CALL_EVENT; trig_EPSS output FUNCTION_CALL_EVENT; trig_OSP output FUNCTION_CALL_EVENT; trig_Hw_Out output FUNCTION_CALL_EVENT; trig_LIDR output FUNCTION_CALL_EVENT; trig_HAL_In output FUNCTION_CALL_EVENT; trig_INP output FUNCTION_CALL_EVENT; trig_APP output FUNCTION_CALL_EVENT; trig_OUTP output FUNCTION_CALL_EVENT

== stateflow chart OSP/OSP/Function Call Generator EPAS2 ==
  (default) -> (junction 81)
  (junction 81) -> (junction 82) [order 1] : [SampleTime_S<=C_TASK_1MS_S]
  (junction 81) -> (junction 83) [order 2] : {Timer=Timer+C_TASK_1MS_S;}
  (junction 82) -> (junction 85) : {FunCall;}
  (junction 83) -> (junction 84) [order 1] : [Timer>=SampleTime_S-0.0001]
  (junction 83) -> (junction 87) [order 2]
  (junction 84) -> (junction 86) : {FunCall;}
  (junction 85) -> (junction 89) : {Timer=0;}
  (junction 86) -> (junction 88) : {Timer=0;}
  (junction 88) -> (junction 87)
  (junction 89) -> (junction 88)
  data: SampleTime_S input double; C_TASK_1MS_S parameter double; Timer local single
  events: FunCall output FUNCTION_CALL_EVENT

== stateflow chart OSP/OSP/Function Call Generator EPAS3 ==
  (default) -> (junction 107)
  (junction 107) -> (junction 108) [order 1] : [SampleTime_S<=C_TASK_1MS_S]
  (junction 107) -> (junction 109) [order 2] : {Timer=Timer+C_TASK_1MS_S;}
  (junction 108) -> (junction 111) : {FunCall;}
  (junction 109) -> (junction 110) [order 1] : [Timer>=SampleTime_S-0.0001]
  (junction 109) -> (junction 113) [order 2]
  (junction 110) -> (junction 112) : {FunCall;}
  (junction 111) -> (junction 115) : {Timer=0;}
  (junction 112) -> (junction 114) : {Timer=0;}
  (junction 114) -> (junction 113)
  (junction 115) -> (junction 114)
  data: SampleTime_S input double; C_TASK_1MS_S parameter double; Timer local single
  events: FunCall output FUNCTION_CALL_EVENT

== stateflow chart EPSS/EPSS/AngleMode/Angle2Torque/Rate_Limit/RateLimiter/Chart ==
  state Increase
    en:
    tou=increase_tou;
    Max=Data_in;
    Min=-10000000000;
    Initial=0;
    du:
    tou=increase_tou;
    Max=Data_in;
    Min=-10000000000;
    Initial=0;
  state Decrease
    en:
    tou=decrease_tou;
    Max=10000000000;
    Min=Data_in;
    Initial=0;
    du:
    tou=decrease_tou;
    Max=10000000000;
    Min=Data_in;
    Initial=0;
  state Start
    en:
    tou=0;
    Max=10000000000;
    Min=-10000000000;
    Initial=1;
  (default) -> Start
  Start -> Increase [order 2] : [increase]
  Start -> Decrease [order 1] : [decrease]
  Increase -> Decrease : [decrease]
  Decrease -> Increase : [increase]
  data: Initial output double; increase input double; decrease input double; Data_in input double; increase_tou input double; decrease_tou input double; tou output double; Min output double; Max output double

== stateflow chart OSP/OSP/Function Call Generator SAS1 ==
  (default) -> (junction 152)
  (junction 152) -> (junction 153) [order 1] : [SampleTime_S<=C_TASK_1MS_S]
  (junction 152) -> (junction 154) [order 2] : {Timer=Timer+C_TASK_1MS_S;}
  (junction 153) -> (junction 156) : {FunCall;}
  (junction 154) -> (junction 155) [order 1] : [Timer>=SampleTime_S-0.0001]
  (junction 154) -> (junction 158) [order 2]
  (junction 155) -> (junction 157) : {FunCall;}
  (junction 156) -> (junction 160) : {Timer=0;}
  (junction 157) -> (junction 159) : {Timer=0;}
  (junction 159) -> (junction 158)
  (junction 160) -> (junction 159)
  data: SampleTime_S input double; C_TASK_1MS_S parameter double; Timer local single
  events: FunCall output FUNCTION_CALL_EVENT

== matlab function dHAL_IN/HAL_IN_RadObjDecoder/RObj_Parser/RObj_FramesParser ==
  data: Frames1 input uint8; Obj_RolCount output uint8; Obj_ID output uint8; Obj_LongDispl output single; Obj_VrelLong output single; Obj_AccelLong output single; Obj_LatDispl output single; Obj_DynProp output uint8; Obj_ProbOfExist output uint8; Obj_MeasStat output uint8; Obj_Width output uint8; Obj_Length output uint8; Frames2 input uint8; Obj_RCSValue output single; Obj_LatSpeed output single; Obj_ObstacleProb output uint8
function [Obj_RolCount,Obj_ID, Obj_LongDispl, Obj_VrelLong, Obj_AccelLong, Obj_LatDispl, Obj_DynProp, Obj_ProbOfExist, Obj_MeasStat, Obj_Width, Obj_Length, Obj_RCSValue, Obj_LatSpeed, Obj_ObstacleProb] = fcn(Frames1, Frames2)

NofObjects = uint8(40);
Obj_RolCount = uint8(zeros(1,40));
Obj_ID = uint8(zeros(1,40));
Obj_LongDispl = single(zeros(1,40));
Obj_VrelLong = single(zeros(1,40));
Obj_AccelLong = single(zeros(1,40));
Obj_LatDispl = single(zeros(1,40));
Obj_ProbOfExist = uint8(zeros(1,40));
Obj_DynProp = uint8(zeros(1,40));
Obj_MeasStat = uint8(zeros(1,40));
Obj_RCSValue = single(zeros(1,40));
Obj_LatSpeed = single(zeros(1,40));
Obj_ObstacleProb = uint8(zeros(1,40));
Obj_Length = uint8(zeros(1,40));
Obj_Width = uint8(zeros(1,40));

%%%%%%%%%%%%%%%%%%%%%%%%%%%%%%%
%%%%%%%%%%%% FRAMES1 %%%%%%%%%%
%%%%%%%%%%%%%%%%%%%%%%%%%%%%%%%

Obj_RollCount_Mask = uint8(bin2dec ('00000011'));
Obj_ID_Mask = uint8(bin2dec('11111100'));
Obj_LongDispl_Mask = uint8(bin2dec('11100000'));
Obj_VrelLong_b1_Mask = uint8(bin2dec('00011111'));
Obj_VrelLong_b2_Mask = uint8(bin2dec('11111110'));
Obj_AccelLong_b1_Mask = uint8(bin2dec('000000001'));
Obj_LatDispl_b2_Mask = uint8(bin2dec('11000000'));
Obj_DynProp_b1_Mask = uint8(bin2dec('00111000'));
Obj_ProbOfExist_b1_Mask = uint8(bin2dec('00000111'));
Obj_MeasStat_b1_Mask = uint8(bin2dec('11000000'));
Obj_Width_b1_Mask = uint8(bin2dec('00111000'));
Obj_Length_b1_Mask = uint8(bin2dec('00000111'));

for Obj_Count = 1:NofObjects

Obj_RolCount(1,Obj_Count) = bitand(uint8(Frames1(1,Obj_Count)),Obj_RollCount_Mask);     
Obj_ID(1,Obj_Count) = bitshift(bitand(Frames1(1,Obj_Count),Obj_ID_Mask),-2);

Obj_LongDispl_2byte = uint16(bitshift(bitand(Frames1(3,Obj_Count),Obj_LongDispl_Mask),-5));
Obj_LongDispl_u16 = uint16(bitshift(uint16(Frames1(2,Obj_Count)),3));
Obj_LongDispl_u16 = uint16(bitor(Obj_LongDispl_u16,Obj_LongDispl_2byte));
Obj_LongDispl(1,Obj_Count) = single(single(Obj_LongDispl_u16)*0.1);

Obj_VrelLong_byte1 = uint16(bitshift(bitand(uint16(Frames1(3,Obj_Count)),uint16(Obj_VrelLong_b1_Mask)),7));
Obj_VrelLong_byte2 = uint16(bitshift(bitand(Frames1(4,Obj_Count),Obj_VrelLong_b2_Mask),-1));
Obj_VrelLong_u16 = uint16(bitor(Obj_VrelLong_byte1,Obj_VrelLong_byte2));
Obj_VrelLong(1,Obj_Count) = single(single(Obj_VrelLong_u16)*0.0625);
Obj_VrelLong(1,Obj_Count) = Obj_VrelLong(1,Obj_Count) - 128;

Obj_AccelLong_byte1 = uint16(bitand(uint16(Frames1(4,Obj_Count)),uint16(Obj_AccelLong_b1_Mask)));
Obj_AccelLong_u16 = uint16(bitor(Obj_AccelLong_byte1,uint16(Frames1(5,Obj_Count))));
Obj_AccelLong(1,Obj_Count) = single(single(Obj_AccelLong_u16)*0.0625);
Obj_AccelLong(1,Obj_Count) = Obj_AccelLong(1,Obj_Count) - 16;


Obj_LatDispl_byte2 = uint16(bitand(uint16(Frames1(7,Obj_Count)),uint16(Obj_LatDispl_b2_Mask)));
Obj_LatDispl_byte2 = bitshift(Obj_LatDispl_byte2,-6);
Obj_LatDispl_byte1 = uint16(bitshift(uint16(Frames1(6,Obj_Count)),2));
Obj_LatDispl_u16 = uint16(bitor(Obj_LatDispl_byte1,Obj_LatDispl_byte2));
Obj_LatDispl(1,Obj_Count) = single(single(Obj_LatDispl_u16) * 0.1);
Obj_LatDispl(1,Obj_Count) = Obj_LatDispl(1,Obj_Count) - 52;

Obj_ProbOfExist(1,Obj_Count) = uint8(bitand(Frames1(7,Obj_Count),Obj_ProbOfExist_b1_Mask));

Obj_DynProp(1,Obj_Count) = uint8(bitand(Frames1(7,Obj_Count),Obj_DynProp_b1_Mask));
Obj_DynProp(1,Obj_Count) = uint8(bitshift(Obj_DynProp(1,Obj_Count),-3));

Obj_Length(1,Obj_Count) = uint8(bitand(Frames1(8,Obj_Count),Obj_Length_b1_Mask));

Obj_Width(1,Obj_Count) = uint8(bitand(Frames1(8,Obj_Count),Obj_Width_b1_Mask));
Obj_Width(1,Obj_Count) = uint8(bitshift(Obj_Width(1,Obj_Count),-3));

Obj_MeasStat(1,Obj_Count) = uint8(bitand(Frames1(8,Obj_Count),Obj_MeasStat_b1_Mask));
Obj_MeasStat(1,Obj_Count) = uint8(bitshift(Obj_MeasStat(1,Obj_Count),-6));

%%%%%%%%%%%%%%%%%%%%%%%%%%%%%%%
%%%%%%%%%%%% FRAMES2 %%%%%%%%%%
%%%%%%%%%%%%%%%%%%%%%%%%%%%%%%%

Obj_ObstacleProb_b1_Mask = uint8(bin2dec('01111111'));

Obj_RCSValue(1,Obj_Count) = (single(Frames2(1,Obj_Count))*0.5)-64;
Obj_LatSpeed(1,Obj_Count) = (single(Frames2(2,Obj_Count))*0.25)-32;
Obj_ObstacleProb(1,Obj_Count) = uint8(bitand(Frames2(3,Obj_Count),Obj_ObstacleProb_b1_Mask));

end

end

== matlab function dHAL_IN/HAL_IN_RadObjDecoder/RObj_Parser/RObj_StatusParser ==
  data: Status_Frame input uint8 size=8; N_of_Objects output uint8; MeasCounter output uint16; SensorRxInvalid output uint8; SensorSupplyVoltage output uint8; SensorDefective output uint8; SensorMisaligned output uint8; SensorSwitchedOff output uint8; SensorExternalDisturbed output uint8; SensorOutputReduced output uint8; LatDistToborderLeft output single; LatDistToborderRight output single
function [N_of_Objects,MeasCounter, SensorRxInvalid, SensorSupplyVoltage, SensorDefective, SensorMisaligned, SensorSwitchedOff, SensorExternalDisturbed, SensorOutputReduced, LatDistToborderLeft, LatDistToborderRight] = fcn(Status_Frame)


N_of_Objects = uint8(Status_Frame(1,1));

MeasCounter = typecast([Status_Frame(2,1) Status_Frame(3,1)],'uint16');   

SensorRxInvalid = bitget(Status_Frame(4,1),7);
SensorSupplyVoltage = bitget(Status_Frame(4,1),6);
SensorDefective = bitget(Status_Frame(4,1),5);
SensorMisaligned = bitget(Status_Frame(4,1),4);
SensorSwitchedOff = bitget(Status_Frame(4,1),3);
SensorExternalDisturbed = bitget(Status_Frame(4,1),2);
SensorOutputReduced = bitget(Status_Frame(4,1),1);
LatDistToborderLeft = single(single(Status_Frame(6,1))*0.1);
LatDistToborderRight = single(single(Status_Frame(7,1))*0.1);



end

== stateflow chart dHAL_IN/HAL_IN_RadObjDecoder/RObjectPackFrame/RObjects_Decoder_v2/CheckIDs/CAN_RAW_Deco ==
  (default) -> (junction 222)
  (junction 222) -> (junction 224) : {
      | R_Objects_out = R_Objects_in;
      | }
  (junction 225) -> (junction 223) [order 1] : [ID == KHAL_MssgIdObjStatus_num]
  (junction 224) -> (junction 225) [order 1] : [Status == TRUE]
  (junction 223) -> (junction 236) : {
      | R_Objects_out.ObS_on = true;
      | R_Objects_out.ObF1_on = false;
      | R_Objects_out.ObF2_on = false;
      | }
  (junction 224) -> (junction 230) [order 2]
  (junction 225) -> (junction 226) [order 2]
  (junction 226) -> (junction 227) [order 1] : [ID == KHAL_MssgIdObj1_num]
  (junction 226) -> (junction 228) [order 2]
  (junction 227) -> (junction 235) : {
      | R_Objects_out.ObS_on = false;
      | R_Objects_out.ObF1_on = true;
      | R_Objects_out.ObF2_on = false;
      | }
  (junction 228) -> (junction 229) : [ID == KHAL_MssgIdObj2_num]
  (junction 229) -> (junction 234) : {
      | R_Objects_out.ObS_on = false;
      | R_Objects_out.ObF1_on = false;
      | R_Objects_out.ObF2_on = true;
      | }
  (junction 230) -> (junction 231) [order 1] : [Status == FALSE]
  (junction 230) -> (junction 232) [order 2]
  (junction 231) -> (junction 233) : {
      | R_Objects_out.ObS_on = false;
      | R_Objects_out.ObF1_on = false;
      | R_Objects_out.ObF2_on = false;
      | }
  (junction 233) -> (junction 232)
  (junction 234) -> (junction 233)
  (junction 235) -> (junction 234)
  (junction 236) -> (junction 235)
  (junction 232) -> (junction 237) : {
      | ParseFrames;
      | }
  (junction 237) -> (junction 238)
  data: Status input boolean; ID input uint32; KHAL_MssgIdObj1_num parameter double; KHAL_MssgIdObj2_num parameter double; KHAL_MssgIdObjStatus_num parameter double; R_Objects_in input Bus: R_Objects; R_Objects_out output Bus: R_Objects; TRUE parameter boolean; FALSE parameter boolean
  events: ParseFrames output FUNCTION_CALL_EVENT

== matlab function dHAL_IN/HAL_IN_RadObjDecoder/RObjectPackFrame/RObjects_Decoder_v2/ParseFrames/MATLAB Function ==
  data: R_Objects_in input Bus: R_Objects; Byte1 input uint8; Byte2 input uint8; Byte3 input uint8; Byte4 input uint8; Byte5 input uint8; Byte6 input uint8; Byte7 input uint8; Byte8 input uint8; R_Objects_out output Bus: R_Objects
function R_Objects_out  = fcn(R_Objects_in, Byte1, Byte2, Byte3, Byte4, Byte5, Byte6, Byte7, Byte8)


R_Objects_out = R_Objects_in;

if (R_Objects_in.ObS_on == true)

R_Objects_out.StatusFrame(1,1) =  uint8(Byte1);
R_Objects_out.StatusFrame(1,2) =  uint8(Byte2);
R_Objects_out.StatusFrame(1,3) =  uint8(Byte3);
R_Objects_out.StatusFrame(1,4) =  uint8(Byte4);
R_Objects_out.StatusFrame(1,5)=   uint8(Byte5);
R_Objects_out.StatusFrame(1,6) =  uint8(Byte6);
R_Objects_out.StatusFrame(1,7) =  uint8(Byte7);
R_Objects_out.StatusFrame(1,8) =  uint8(Byte8);

R_Objects_out.received_frames1 = uint8(0);
R_Objects_out.received_frames2 = uint8(0);
R_Objects_out.isComplete = false;

elseif (R_Objects_in.ObF1_on == true)

R_Objects_out.received_frames1 = R_Objects_in.received_frames1+1;

R_Objects_out.Frames1(1,R_Objects_out.received_frames1) =  uint8(Byte1);
R_Objects_out.Frames1(2,R_Objects_out.received_frames1) =  uint8(Byte2);
R_Objects_out.Frames1(3,R_Objects_out.received_frames1) =  uint8(Byte3);
R_Objects_out.Frames1(4,R_Objects_out.received_frames1) =  uint8(Byte4);
R_Objects_out.Frames1(5,R_Objects_out.received_frames1)=   uint8(Byte5);
R_Objects_out.Frames1(6,R_Objects_out.received_frames1) =  uint8(Byte6);
R_Objects_out.Frames1(7,R_Objects_out.received_frames1) =  uint8(Byte7);
R_Objects_out.Frames1(8,R_Objects_out.received_frames1) =  uint8(Byte8);


elseif (R_Objects_in.ObF2_on == true)

R_Objects_out.received_frames2 = R_Objects_in.received_frames2+1;

R_Objects_out.Frames2(1,R_Objects_out.received_frames2) =  uint8(Byte1);
R_Objects_out.Frames2(2,R_Objects_out.received_frames2) =  uint8(Byte2);
R_Objects_out.Frames2(3,R_Objects_out.received_frames2) =  uint8(Byte3);
R_Objects_out.Frames2(4,R_Objects_out.received_frames2) =  uint8(Byte4);
R_Objects_out.Frames2(5,R_Objects_out.received_frames2)=   uint8(Byte5);
R_Objects_out.Frames2(6,R_Objects_out.received_frames2) =  uint8(Byte6);
R_Objects_out.Frames2(7,R_Objects_out.received_frames2) =  uint8(Byte7);
R_Objects_out.Frames2(8,R_Objects_out.received_frames2) =  uint8(Byte8);

elseif (R_Objects_out.received_frames1 == 40 && R_Objects_out.received_frames2 == 40)
  
    R_Objects_out.isComplete = true;
    

elseif (R_Objects_in.ObS_on == false && R_Objects_in.ObF2_on == false && R_Objects_in.ObF2_on == false)

    R_Objects_out = R_Objects_in;
    
end


end
